simulink model "ACSwt_VD"  (R2016b)
settings: configuration reference "CodeGenConfigSet" (kept outside this file)
values from neighbouring files (symbols this model uses):
  AirC_stSwtDfl_C = Calibration.Parameter    [init_ACSwt_VD.m]    (also in init_ACSwt_VD_SIL.m = Simulink.Parameter)
  AirC_swtMnSwtSig_C = Calibration.Parameter    [init_ACSwt_VD.m]    (also in init_ACSwt_VD_SIL.m = Simulink.Parameter)
  SigTst_stAirCSwtPrs_C = Calibration.Parameter    [init_ACSwt_VD.m]    (also in init_ACSwt_VD_SIL.m = Simulink.Parameter)
  SigTst_swtAirCSwtPrs_C = Calibration.Parameter    [init_ACSwt_VD.m]    (also in init_ACSwt_VD_SIL.m = Simulink.Parameter)
undefined symbols (not defined in the file or in its folder): Switch_conv
settings Model: Creator=胡炎林  LastModifiedBy=胡炎林
settings ConfigSetRef: SourceLocation=Base Workspace

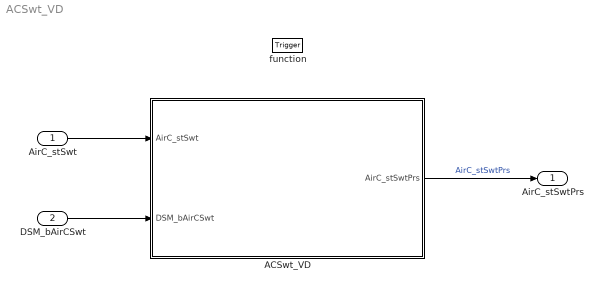
== system ACSwt_VD ==
  AirC_stSwt : Inport  Description=Status of AC switch  OutMin=0  OutMax=1  OutDataTypeStr=boolean
  DSM_bAirCSwt : Inport  Description=state of FId_AirCSwt  Port=2  OutMin=0  OutMax=1  OutDataTypeStr=boolean
  function : TriggerPort  TriggerType=function-call  VariantControl=Variant
  ACSwt_VD : Subsystem  TreatAsAtomicUnit=on  RTWFcnName=ACSwt_VD_Co  RTWFileName=AirC
      settings: RTWSystemCode=Nonreusable function  RTWFcnNameOpts=User specified  RTWFileNameOpts=User specified
  AirC_stSwtPrs : Outport  Description=AC switch pressed/unpressed status  OutMin=0  OutMax=1  OutDataTypeStr=boolean
  wires:
  DSM_bAirCSwt/1 -> ACSwt_VD/2(DSM_bAirCSwt)
  AirC_stSwt/1 -> ACSwt_VD/1(" AirC_stSwt")
  ACSwt_VD/1(" AirC_stSwtPrs") -> AirC_stSwtPrs/1  "AirC_stSwtPrs"

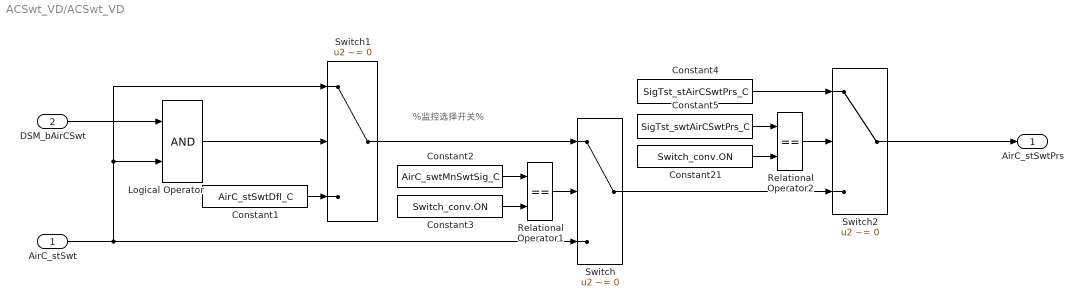
== system ACSwt_VD/ACSwt_VD ==
  note: %监控选择开关%
  " AirC_stSwt" : Inport
  DSM_bAirCSwt : Inport  Port=2
  Constant1 : Constant  Value=AirC_stSwtDfl_C
  Constant2 : Constant  Value=AirC_swtMnSwtSig_C
  Constant21 : Constant  Value=Switch_conv.ON  OutDataTypeStr=Inherit: Inherit via back propagation
  Constant3 : Constant  Value=Switch_conv.ON  OutDataTypeStr=Inherit: Inherit via back propagation
  Constant4 : Constant  Value=SigTst_stAirCSwtPrs_C
  Constant5 : Constant  Value=SigTst_swtAirCSwtPrs_C
  Logical Operator : Logic  OutDataTypeStr=boolean
  Relational Operator1 : RelationalOperator  Operator===  OutDataTypeStr=boolean  RndMeth=Simplest  InputSameDT=on
  Relational Operator2 : RelationalOperator  Operator===  OutDataTypeStr=boolean  RndMeth=Simplest  InputSameDT=on
  Switch : Switch  Criteria=u2 ~= 0  InputSameDT=on
  Switch1 : Switch  Criteria=u2 ~= 0  InputSameDT=on
  Switch2 : Switch  Criteria=u2 ~= 0  InputSameDT=on
  " AirC_stSwtPrs" : Outport
  wires:
  Constant1/1 -> Switch1/3
  Switch2/1 -> " AirC_stSwtPrs"/1
  Logical Operator/1 -> Switch1/2
  Switch1/1 -> Switch/1
  Relational Operator1/1 -> Switch/2
  " AirC_stSwt"/1 -> Switch1/1, Logical Operator/2, Switch/3
  Constant2/1 -> Relational Operator1/1
  Constant3/1 -> Relational Operator1/2
  Constant5/1 -> Relational Operator2/1
  Constant4/1 -> Switch2/1
  Constant21/1 -> Relational Operator2/2
  Relational Operator2/1 -> Switch2/2
  Switch/1 -> Switch2/3
  DSM_bAirCSwt/1 -> Logical Operator/1
